simulink model "smc02"  (R2024a)
settings: Solver=VariableStepAuto  StartTime=0.0  StopTime=10.0  RelTol=1e-3
libraries: spspowerguiLib x1
settings Model: Creator=XieXW  LastModifiedBy=XieXW
settings SolverCC: ZeroCrossAlgorithm=Adaptive
settings DebuggingCC: IgnoredZcDiagnostic=none

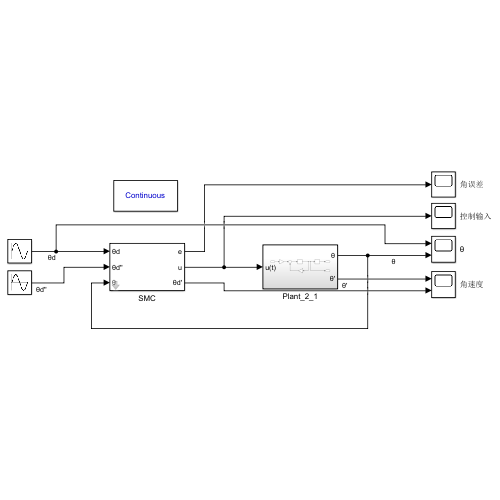
[thumbnail: Simulink's stored preview of the top-level diagram]
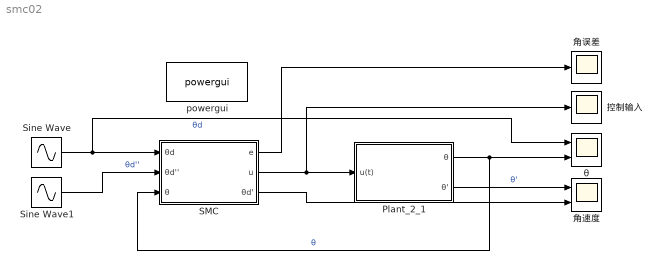
== system smc02 ==
  Plant_2_1 : Subsystem
  SMC : Subsystem  mask{c=15, k=10, epsilon=5}
      mask prompts: c "滑模增益c"; k "趋近速度k"; epsilon "ε"
      mask DialogControl ParameterGroupVar Prompt: 参数
  Sine Wave : Sin  SampleTime=0
  Sine Wave1 : Sin  Phase=pi  SampleTime=0
  powergui : spspowerguiLib/powergui  Priority=1  SimulationMode=Continuous  SampleTime=50e-6  frequency=60  Iterations=50  frequencyindice=60  Pbase=100e6  ErrMax=1e-4  UnitsV=kV  UnitsW=MW  buscounter=0  FunctionMessages=off  echomessages=off  EnableUseOfTLC=off  CurrentSourceSwitches=off  DisableSnubberDevices=off  DisableRonSwitches=off  DisableVfSwitches=off  DisplayEquations=off  AutomaticDiscreteSolvers=off  SolverType=Tustin/Backward Euler (TBE)  Interpol=off  ExternalGateDelay=off  methode=off  Ts=100  x0status=blocks  SPID=on  SwTol=0  HookPort=off  NonlinearTolerance=1e-4  nMaxIteration=100  ContinueOnMaxIteration=off  RestoreLinks=warning  ResistiveCurrentMeasurement=off  Frange=[0:2:500]  Ylog=off  Xlog=on  ShowGrid=off  save=off  variable=ZData  structure=0  ZoomFFT=off  StartTime=0.0  cycles=1  DisplayStyle=1  fundamental=60  FreqAxis=off  MaxFrequency=1000  frequencyindicesteady=1  RmsSteady=1  display=off
  θ : Scope  NumInputPorts=2
  控制输入 : Scope
  角误差 : Scope
  角速度 : Scope  NumInputPorts=2
  wires:
  Sine Wave/1 -> θ/1, SMC/1(θd)  "θd"
  Plant_2_1/1(θ) -> SMC/3(θ), θ/2  "θ"
  Sine Wave1/1 -> SMC/2(θd'')  "θd''"
  SMC/2(u) -> 控制输入/1, Plant_2_1/1(u(t))
  SMC/1(e) -> 角误差/1
  Plant_2_1/2(θ') -> 角速度/1  "θ'"
  SMC/3(θd') -> 角速度/2

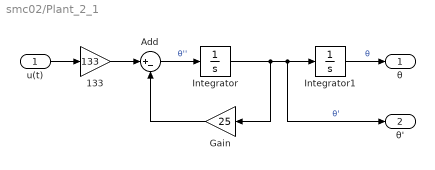
== system smc02/Plant_2_1 ==
  u(t) : Inport
  133 : Gain  Gain=133
  Add : Sum  Inputs=|+-
  Gain : Gain  Gain=25
  Integrator : Integrator
  Integrator1 : Integrator
  θ : Outport
  θ' : Outport  Port=2
  wires:
  u(t)/1 -> 133/1
  133/1 -> Add/1
  Integrator/1 -> Gain/1, Integrator1/1, θ'/1  "θ'"
  Add/1 -> Integrator/1  "θ''"
  Gain/1 -> Add/2
  Integrator1/1 -> θ/1  "θ"

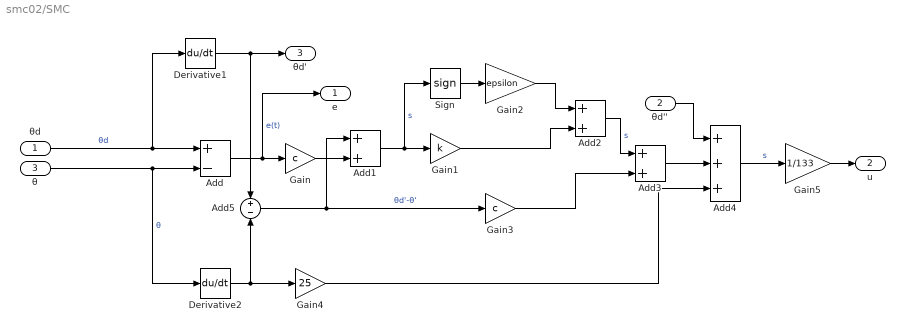
== system smc02/SMC ==
  θd : Inport
  θd'' : Inport  Port=2
  θ : Inport  Port=3
  Add : Sum  Inputs=+-
  Add1 : Sum
  Add2 : Sum
  Add3 : Sum
  Add4 : Sum  Inputs=+++
  Add5 : Sum  Inputs=+-
  Derivative1 : Derivative
  Derivative2 : Derivative
  Gain : Gain  Gain=c
  Gain1 : Gain  Gain=k
  Gain2 : Gain  Gain=epsilon
  Gain3 : Gain  Gain=c
  Gain4 : Gain  Gain=25
  Gain5 : Gain  Gain=1/133
  Sign : Signum
  e : Outport
  u : Outport  Port=2
  θd' : Outport  Port=3
  wires:
  θd/1 -> Derivative1/1, Add/1  "θd"
  θ/1 -> Derivative2/1, Add/2  "θ"
  Add/1 -> e/1, Gain/1  "e(t)"
  Gain/1 -> Add1/2
  Add1/1 -> Sign/1, Gain1/1  "s"
  Sign/1 -> Gain2/1
  Gain2/1 -> Add2/1
  Gain1/1 -> Add2/2
  Gain3/1 -> Add3/2
  Add2/1 -> Add3/1  "s"
  Derivative2/1 -> Gain4/1, Add5/2
  Derivative1/1 -> θd'/1, Add5/1
  Add3/1 -> Add4/2
  Gain4/1 -> Add4/3
  Add4/1 -> Gain5/1  "s"
  Gain5/1 -> u/1
  Add5/1 -> Gain3/1, Add1/1  "θd'-θ‘"
  θd''/1 -> Add4/1
